simulink model "JacobiansTest"  (Simulink 7.9)
settings: Solver=ode45  StartTime=0.0  StopTime=inf  RelTol=1e-3
undefined symbols (not defined in the file or in its folder): qinit
libraries: utility x1, dspmtrx3 x1
settings Model: Creator=jorhabib  LastModifiedBy=jorhabib

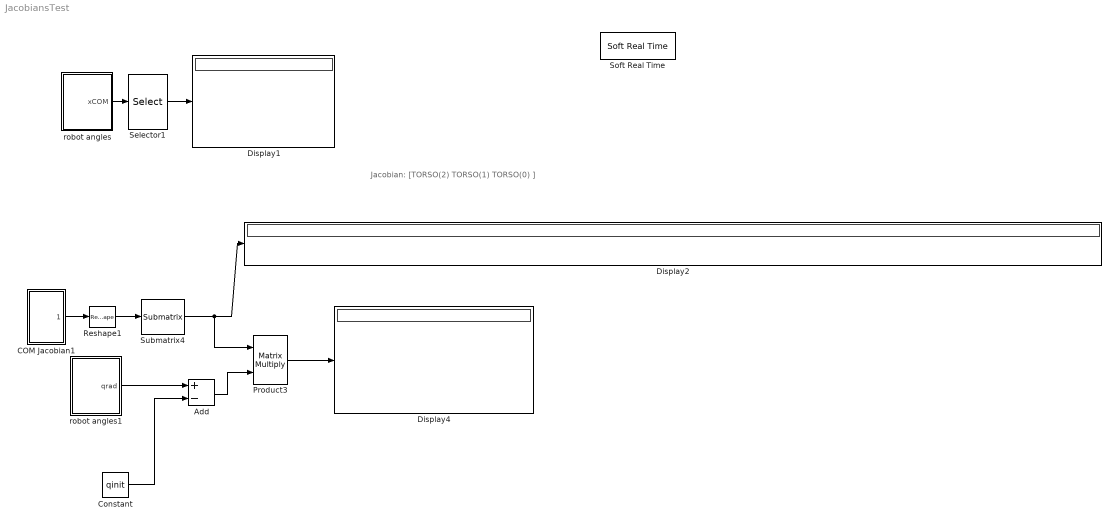
== system JacobiansTest ==
  note: Jacobian: [TORSO(2) TORSO(1) TORSO(0) ]
  Add : Sum  Inputs=+-
  COM Jacobian1 : Subsystem
  Constant : Constant  Value=qinit
  Display1 : Display
  Display2 : Display
  Display4 : Display
  Product3 : Product  Multiplication=Matrix(*)  RndMeth=Zero
  Reshape1 : Reshape  OutputDimensionality=Customize  OutputDimensions=[6,31]
  Selector1 : Selector  IndexMode=Zero-based  InputPortWidth=7  IndexOptions=Index vector (dialog)  Indices=[0:1]  OutputSizes=1
  Soft Real Time : utility/Soft Real Time  x=0.02
  Submatrix4 : dspmtrx3/Submatrix  RowSpan=Range of rows  RowStartMode=First  RowStartIndex=1  RowEndMode=Index  RowEndIndex=2  ColSpan=Range of columns  ColStartMode=Index  ColStartIndex=7  ColEndMode=Last  ColEndIndex=6
  robot angles : Subsystem
  robot angles1 : Subsystem
  wires:
  COM Jacobian1/1(Jacobian) -> Reshape1/1
  Reshape1/1 -> Submatrix4/1
  Submatrix4/1 -> Display2/1, Product3/1
  robot angles/1(xCOM) -> Selector1/1
  Selector1/1 -> Display1/1
  Product3/1 -> Display4/1
  robot angles1/1(qrad) -> Add/1
  Add/1 -> Product3/2
  Constant/1 -> Add/2

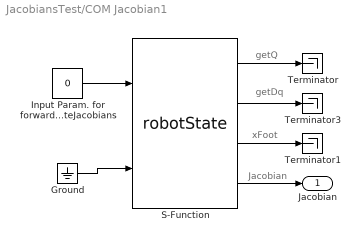
== system JacobiansTest/COM Jacobian1 ==
  note: Jacobian
  note: getQ
  note: xFoot
  note: getDq
  Ground : Ground
  "Input Param. for forwardKinematics and  computeJacobians " : Constant  Value=0  OutDataTypeStr=int8
  S-Function : S-Function  FunctionName=robotState  Parameters=val,robotname,localname  EnableBusSupport=off  mask{val=3, robotname='icubSim', localname='robotState'}
      mask prompts: val "Value"; robotname "Robot Name (icub - icubSim)"; localname "Module Name"
  Terminator : Terminator
  Terminator1 : Terminator
  Terminator3 : Terminator
  Jacobian : Outport
  wires:
  S-Function/4 -> Jacobian/1
  "Input Param. for forwardKinematics and  computeJacobians "/1 -> S-Function/1
  S-Function/3 -> Terminator1/1
  S-Function/1 -> Terminator/1
  S-Function/2 -> Terminator3/1
  Ground/1 -> S-Function/2

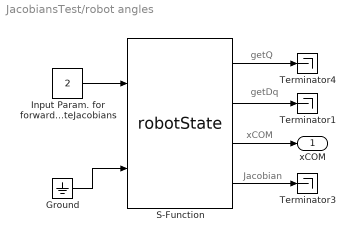
== system JacobiansTest/robot angles ==
  note: Jacobian
  note: getQ
  note: xCOM
  note: getDq
  Ground : Ground
  "Input Param. for forwardKinematics and  computeJacobians " : Constant  Value=2  OutDataTypeStr=int8
  S-Function : S-Function  FunctionName=robotState  Parameters=val,robotname,localname  EnableBusSupport=off  mask{val=2, robotname='icubSim', localname='robotState'}
      mask prompts: val "Value"; robotname "Robot Name (icub - icubSim)"; localname "Module Name"
  Terminator1 : Terminator
  Terminator3 : Terminator
  Terminator4 : Terminator
  xCOM : Outport
  wires:
  S-Function/4 -> Terminator3/1
  "Input Param. for forwardKinematics and  computeJacobians "/1 -> S-Function/1
  S-Function/3 -> xCOM/1
  S-Function/1 -> Terminator4/1
  S-Function/2 -> Terminator1/1
  Ground/1 -> S-Function/2

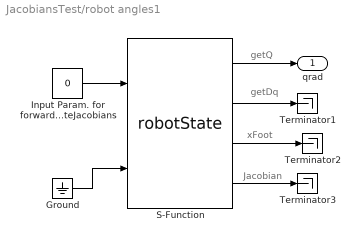
== system JacobiansTest/robot angles1 ==
  note: getDq
  note: xFoot
  note: getQ
  note: Jacobian
  Ground : Ground
  "Input Param. for forwardKinematics and  computeJacobians " : Constant  Value=0  OutDataTypeStr=int8
  S-Function : S-Function  FunctionName=robotState  Parameters=val,robotname,localname  EnableBusSupport=off  mask{val=0, robotname='icubSim', localname='robotState'}
      mask prompts: val "Value"; robotname "Robot Name (icub - icubSim)"; localname "Module Name"
  Terminator1 : Terminator
  Terminator2 : Terminator
  Terminator3 : Terminator
  qrad : Outport
  wires:
  Ground/1 -> S-Function/2
  S-Function/2 -> Terminator1/1
  S-Function/1 -> qrad/1
  S-Function/3 -> Terminator2/1
  "Input Param. for forwardKinematics and  computeJacobians "/1 -> S-Function/1
  S-Function/4 -> Terminator3/1
